simulink model "Copy_of_minimal_rcu_full"  (R2014b)
settings: Solver=ode4  SolverMode=SingleTasking  StartTime=0.0  StopTime=t_sim  FixedStep=sample_time_model  RelTol=1e-3
PreLoadFcn:
  | initModell
InitFcn:
  | initModell
undefined symbols (not defined in the file): FILTER_TAU_EXT, FIXED_FILTER_BANDWIDTH, FIXED_FILTER_BANDWIDTH_OBSERVER, iter, K_INV, KI2TAU_VEC, KS_trq, KT_trq, load_inertia, load_mass, MAX_CURRENT, MIN_SING_VALUE_M_CART, q0, rCEE_i, sample_time_model, sample_time_robot, tau_max
libraries: simulink x69, robotics x15, beasty_sfcns x7, lwr_dynamics x6, trafo3dLib x4, holgersRobLib x3, dspmtrx3 x1, dspinverses x1
(part 4 of 4)

== system Copy_of_minimal_rcu_full/Roboter+controller/controller/Cartesian Impedance Control/Subsystem/Cartesian Compliance Control/Iterative Computation of the 'Stiffness' and Gravity Compensation/Iteration for Nolcos Controller/Spatial Stiffness ==
  Hsd : Inport
  Fkin : Inport  Port=2
  Jbody : Inport  Port=3
  K : Inport  Port=4
  relaxing : Inport  Port=5
  Enable : EnablePort  StatesWhenEnabling=reset
  Kc : Selector  NumberOfDimensions=2  InputPortWidth=3  IndexOptions=Index vector (dialog),Index vector (dialog)  Indices=1:3,4:6
  Kr : Selector  NumberOfDimensions=2  InputPortWidth=3  IndexOptions=Index vector (dialog),Index vector (dialog)  Indices=4:6,4:6
  Kt : Selector  NumberOfDimensions=2  InputPortWidth=3  IndexOptions=Index vector (dialog),Index vector (dialog)  Indices=1:3,1:3
  Math Function : Math  Operator=transpose  SaturateOnIntegerOverflow=on
  Product2 : Product  RndMeth=Zero
  Product4 : Product  Multiplication=Matrix(*)  RndMeth=Zero
  Reshape1 : Reshape
  Reshape2 : Reshape
  Reshape3 : Reshape  OutputDimensionality=Column vector (2-D)
  Spatial Stiffness with varying length and varying stiffness : Subsystem  AncestorBlock=|
      | robotics/Spatial Stiffness
      | with varying length
      | and varying stiffness
  Terminator : Terminator
  Trafo3D Inverse : robotics/Trafo3D Inverse
  Trafo3D Mult : robotics/Trafo3D Mult
  unit frame : Constant  Value=[eye(3),[0;0;0]]
  tau : Outport
  J : Outport  Port=2
  F : Outport  Port=3
  wires:
  Product4/1 -> Reshape2/1
  Jbody/1 -> J/1, Math Function/1
  Math Function/1 -> Product4/1
  Hsd/1 -> Trafo3D Inverse/1
  Trafo3D Inverse/1 -> Trafo3D Mult/1
  Fkin/1 -> Trafo3D Mult/2
  Trafo3D Mult/1 -> Spatial Stiffness with varying length and varying stiffness/1(H12)
  unit frame/1 -> Spatial Stiffness with varying length and varying stiffness/2(H1,1c), Spatial Stiffness with varying length and varying stiffness/3(H2,2c)
  Spatial Stiffness with varying length and varying stiffness/2(W2) -> Product2/1, Reshape1/1
  K/1 -> Kt/1, Kr/1, Kc/1
  Kt/1 -> Spatial Stiffness with varying length and varying stiffness/4(Kt)
  Kr/1 -> Spatial Stiffness with varying length and varying stiffness/5(Kr)
  Kc/1 -> Spatial Stiffness with varying length and varying stiffness/6(Kc)
  relaxing/1 -> Reshape3/1
  Product2/1 -> Product4/2
  Spatial Stiffness with varying length and varying stiffness/1(W1) -> Terminator/1
  Reshape1/1 -> F/1
  Reshape2/1 -> tau/1
  Reshape3/1 -> Product2/2

== system Copy_of_minimal_rcu_full/Roboter+controller/controller/Cartesian Impedance Control/Subsystem/Cartesian Compliance Control/Nullspace Stiffness1/Stiffness Calculation/Calculate reflected Inertia ==
  B_JT_4 : Inport
  0_T_4 : Inport  Port=2
  Mass : Inport  Port=3
  Math Function1 : Math  Operator=transpose  SaturateOnIntegerOverflow=on
  Product : Product  Multiplication=Matrix(*)  RndMeth=Zero
  Product1 : Product  Inputs=3  Multiplication=Matrix(*)  RndMeth=Zero
  Selector translation1 : Selector  NumberOfDimensions=2  InputPortWidth=6  IndexOptions=Index vector (dialog),Index vector (dialog)  Indices=3,3  OutputSizes=1,1
  Trafo3D Adjoint : trafo3dLib/Trafo3D Adjoint
  m_z : Outport
  wires:
  Selector translation1/1 -> m_z/1
  Trafo3D Adjoint/1 -> Product/2
  Math Function1/1 -> Product1/1
  Product/1 -> Product1/3, Math Function1/1
  Product1/1 -> Selector translation1/1
  Mass/1 -> Product1/2
  B_JT_4/1 -> Product/1
  0_T_4/1 -> Trafo3D Adjoint/1

== system Copy_of_minimal_rcu_full/Roboter+controller/controller/Cartesian Impedance Control/Subsystem/Cartesian Compliance Control/Nullspace Stiffness1/Stiffness Calculation/Normalize Vector ==
  In1 : Inport
  Constant : Constant
  Demux : Demux  Outputs=[-1 1]
  Divide : Product  Inputs=*/
  Ground : Ground
  Math Function : Math  Operator=square  SaturateOnIntegerOverflow=on
  Math Function1 : Math  Operator=sqrt  SaturateOnIntegerOverflow=on
  Mux : Mux  Inputs=2
  Mux1 : Mux  Inputs=2
  Product : Product  RndMeth=Zero
  Sum of Elements : Sum  Inputs=+
  Switch : Switch  Criteria=u2 > Threshold  Threshold=maxzero
  Out1 : Outport
  wires:
  Ground/1 -> Product/2
  Product/1 -> Mux1/1
  Constant/1 -> Mux1/2
  Mux1/1 -> Switch/3
  Sum of Elements/1 -> Math Function1/1
  Math Function/1 -> Sum of Elements/1
  Demux/2 -> Divide/2
  Demux/1 -> Divide/1
  Switch/1 -> Demux/1
  Mux/1 -> Switch/1
  Math Function1/1 -> Mux/2, Switch/2
  In1/1 -> Product/1, Math Function/1, Mux/1
  Divide/1 -> Out1/1

== system Copy_of_minimal_rcu_full/Roboter+controller/controller/Cartesian Impedance Control/Subsystem/Cartesian Compliance Control/Nullspace Stiffness1/Stiffness Calculation/PT1_1 ==
  In1 : Inport
  Gain : Gain  Gain=3
  Integrator : Integrator  InitialCondition=[0 0 0]'
  Sum : Sum  Inputs=|+-
  Out1 : Outport  OutDataTypeStr=double  PortDimensions=[3 1]
  wires:
  Integrator/1 -> Sum/2, Out1/1
  Sum/1 -> Gain/1
  In1/1 -> Sum/1
  Gain/1 -> Integrator/1

== system Copy_of_minimal_rcu_full/Roboter+controller/controller/Cartesian Impedance Control/Subsystem/Cartesian Compliance Control/Nullspace Stiffness1/Stiffness Calculation/PT1_2 ==
  In1 : Inport
  Gain : Gain  Gain=3
  Integrator : Integrator
  Sum : Sum  Inputs=|+-
  Out1 : Outport  OutDataTypeStr=double  PortDimensions=1
  wires:
  Gain/1 -> Integrator/1
  In1/1 -> Sum/1
  Sum/1 -> Gain/1
  Integrator/1 -> Sum/2, Out1/1

== system Copy_of_minimal_rcu_full/Roboter+controller/controller/Joint Impedance/JOINT_IMPEDANCE_CONTROL/Joint Compliance Control/Damping Design via Generalized Eigenvalues/Damping Design via Generalized Eigenvalues QR right/Subsystem ==
  A : Inport
  B : Inport  Port=2
  Double diagonalization1 : MATLAB Function  TreatAsAtomicUnit=on
  V : Outport
  lambda : Outport  Port=2
  Vinv : Outport  Port=3
  wires:
  A/1 -> Double diagonalization1/1(A)
  B/1 -> Double diagonalization1/2(B)
  Double diagonalization1/3(lambda) -> lambda/1
  Double diagonalization1/2(Vinv) -> Vinv/1
  Double diagonalization1/1(V) -> V/1

== system Copy_of_minimal_rcu_full/Roboter+controller/controller/Cartesian Impedance Control/Subsystem/Cartesian Compliance Control/Iterative Computation of the 'Stiffness' and Gravity Compensation/Iteration for Nolcos Controller/Euler Angle Stiffness/Euler Angle Components ==
  Hsd : Inport
  Fkin : Inport  Port=2
  J : Inport  Port=3
  Cross-Product : robotics/Cross-Product
  Euler Transf. w->rpy' : robotics/Euler Transf. w->rpy'
  Jv : Selector  NumberOfDimensions=2  InputPortWidth=3  IndexOptions=Index vector (dialog),Select all  Indices=[1 2 3],-1
  Jw : Selector  NumberOfDimensions=2  InputPortWidth=3  IndexOptions=Index vector (dialog),Select all  Indices=[4 5 6],-1
  Matrix Concatenation1 : Concatenate  Mode=Multidimensional array
  Matrix Gain : Gain  Gain=-1  Multiplication=Matrix(K*u)  SaturateOnIntegerOverflow=on  OutDataTypeStr=Inherit: Same as input  ParamDataTypeStr=Inherit: Same as input
  Product1 : Product  Multiplication=Matrix(*)  RndMeth=Zero
  RPY Euler : robotics/RPY Euler  th=0.9999
  Stop Simulation1 : Stop
  Sum3 : Sum  Inputs=-+|  SaturateOnIntegerOverflow=on  InputSameDT=on  OutDataTypeStr=Inherit: Same as first input
  Trafo3D Inverse1 : robotics/Trafo3D Inverse
  Trafo3D Mult1 : robotics/Trafo3D Mult
  v : Selector  NumberOfDimensions=2  InputPortWidth=3  IndexOptions=Select all,Index vector (dialog)  Indices=-1,[4]
  x : Outport
  Jx : Outport  Port=2
  wires:
  Trafo3D Inverse1/1 -> Trafo3D Mult1/1
  Trafo3D Mult1/1 -> RPY Euler/1, v/1
  RPY Euler/2 -> Stop Simulation1/1
  RPY Euler/1 -> Euler Transf. w->rpy'/1, x/1
  v/1 -> Cross-Product/1
  Fkin/1 -> Trafo3D Inverse1/1
  Hsd/1 -> Trafo3D Mult1/2
  J/1 -> Jv/1, Jw/1
  Jw/1 -> Cross-Product/2, Matrix Gain/1
  Sum3/1 -> Matrix Concatenation1/1
  Cross-Product/1 -> Sum3/2
  Jv/1 -> Sum3/1
  Matrix Gain/1 -> Matrix Concatenation1/2
  Matrix Concatenation1/1 -> Product1/2
  Product1/1 -> Jx/1
  Euler Transf. w->rpy'/1 -> Product1/1

== system Copy_of_minimal_rcu_full/Roboter+controller/controller/Cartesian Impedance Control/Subsystem/Cartesian Compliance Control/Iterative Computation of the 'Stiffness' and Gravity Compensation/Iteration for Nolcos Controller/Spatial Stiffness/Spatial Stiffness with varying length and varying stiffness ==
  H12 : Inport
  H1,1c : Inport  Port=2
  H2,2c : Inport  Port=3
  Kt : Inport  Port=4
  Kr : Inport  Port=5
  Kc : Inport  Port=6
  Math Function : Math  Operator=transpose  SaturateOnIntegerOverflow=on
  Math Function1 : Math  Operator=transpose  SaturateOnIntegerOverflow=on
  Product : Product  Multiplication=Matrix(*)  RndMeth=Zero
  Product1 : Product  Multiplication=Matrix(*)  RndMeth=Zero
  Spatial Stiffness without connection offsets : Subsystem
  Trafo3D Adjoint : robotics/Trafo3D Adjoint
  Trafo3D Adjoint1 : robotics/Trafo3D Adjoint
  Trafo3D Inverse : robotics/Trafo3D Inverse
  Trafo3D Inverse1 : robotics/Trafo3D Inverse
  Trafo3D Mult : robotics/Trafo3D Mult
  Trafo3D Mult1 : robotics/Trafo3D Mult
  W1 : Outport
  W2 : Outport  Port=2
  wires:
  Kc/1 -> Spatial Stiffness without connection offsets/4(Kc)
  Kr/1 -> Spatial Stiffness without connection offsets/3(Kr)
  Kt/1 -> Spatial Stiffness without connection offsets/2(Kt)
  Product1/1 -> W2/1
  Spatial Stiffness without connection offsets/2(W2c) -> Product1/2
  Product/1 -> W1/1
  Spatial Stiffness without connection offsets/1(W1c) -> Product/2
  Trafo3D Mult1/1 -> Spatial Stiffness without connection offsets/1(H1c2c)
  H12/1 -> Trafo3D Mult/2
  Trafo3D Mult/1 -> Trafo3D Mult1/1
  Trafo3D Adjoint/1 -> Math Function/1  "AdH1c,1"
  Trafo3D Adjoint1/1 -> Math Function1/1  "AdH2c,2"
  Math Function/1 -> Product/1
  Math Function1/1 -> Product1/1
  H1,1c/1 -> Trafo3D Inverse/1
  Trafo3D Inverse/1 -> Trafo3D Mult/1, Trafo3D Adjoint/1  "H1c,1"
  H2,2c/1 -> Trafo3D Mult1/2, Trafo3D Inverse1/1
  Trafo3D Inverse1/1 -> Trafo3D Adjoint1/1

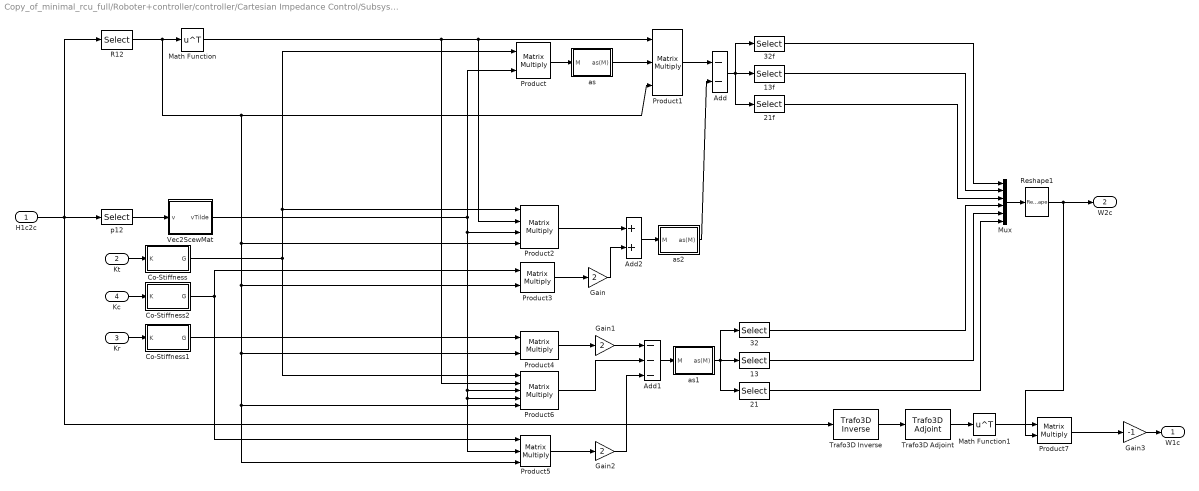
== system Copy_of_minimal_rcu_full/Roboter+controller/controller/Cartesian Impedance Control/Subsystem/Cartesian Compliance Control/Iterative Computation of the 'Stiffness' and Gravity Compensation/Iteration for Nolcos Controller/Spatial Stiffness/Spatial Stiffness with varying length and varying stiffness/Spatial Stiffness without connection offsets ==
  H1c2c : Inport
  Kt : Inport  Port=2
  Kr : Inport  Port=3
  Kc : Inport  Port=4
  13 : Selector  NumberOfDimensions=2  InputPortWidth=3  IndexOptions=Index vector (dialog),Index vector (dialog)  Indices=[1],[3]
  13f : Selector  NumberOfDimensions=2  InputPortWidth=3  IndexOptions=Index vector (dialog),Index vector (dialog)  Indices=[1],[3]
  21 : Selector  NumberOfDimensions=2  InputPortWidth=3  IndexOptions=Index vector (dialog),Index vector (dialog)  Indices=[2],[1]
  21f : Selector  NumberOfDimensions=2  InputPortWidth=3  IndexOptions=Index vector (dialog),Index vector (dialog)  Indices=[2],[1]
  32 : Selector  NumberOfDimensions=2  InputPortWidth=3  IndexOptions=Index vector (dialog),Index vector (dialog)  Indices=[3],[2]
  32f : Selector  NumberOfDimensions=2  InputPortWidth=3  IndexOptions=Index vector (dialog),Index vector (dialog)  Indices=[3],[2]
  Add : Sum  Inputs=--
  Add1 : Sum  Inputs=---
  Add2 : Sum
  Co-Stiffness : Subsystem
  Co-Stiffness1 : Subsystem
  Co-Stiffness2 : Subsystem
  Gain : Gain  Gain=2
  Gain1 : Gain  Gain=2
  Gain2 : Gain  Gain=2
  Gain3 : Gain  Gain=-1
  Math Function : Math  Operator=transpose  SaturateOnIntegerOverflow=on
  Math Function1 : Math  Operator=transpose  SaturateOnIntegerOverflow=on
  Mux : Mux  Inputs=6
  Product{,3..4,7} (4 alike) : Product  Multiplication=Matrix(*)  SaturateOnIntegerOverflow=on  InputSameDT=on  OutDataTypeStr=Inherit: Same as first input
  Product1 : Product  Inputs=3  Multiplication=Matrix(*)  SaturateOnIntegerOverflow=on  InputSameDT=on  OutDataTypeStr=Inherit: Same as first input
  Product2 : Product  Inputs=4  Multiplication=Matrix(*)  SaturateOnIntegerOverflow=on  InputSameDT=on  OutDataTypeStr=Inherit: Same as first input
  Product5 : Product  Inputs=3  Multiplication=Matrix(*)  SaturateOnIntegerOverflow=on  InputSameDT=on  OutDataTypeStr=Inherit: Same as first input
  Product6 : Product  Inputs=5  Multiplication=Matrix(*)  SaturateOnIntegerOverflow=on  InputSameDT=on  OutDataTypeStr=Inherit: Same as first input
  R12 : Selector  NumberOfDimensions=2  InputPortWidth=3  IndexOptions=Index vector (dialog),Index vector (dialog)  Indices=[1,2,3],[1,2,3]
  Reshape1 : Reshape  OutputDimensionality=Column vector (2-D)
  Trafo3D Adjoint : robotics/Trafo3D Adjoint
  Trafo3D Inverse : robotics/Trafo3D Inverse
  Vec2ScewMat : Subsystem
  as : Subsystem
  as1 : Subsystem
  as2 : Subsystem
  p12 : Selector  NumberOfDimensions=2  InputPortWidth=3  IndexOptions=Index vector (dialog),Index vector (dialog)  Indices=[1,2,3],[4]
  W1c : Outport
  W2c : Outport  Port=2
  wires:
  H1c2c/1 -> p12/1, R12/1, Trafo3D Inverse/1
  Kc/1 -> Co-Stiffness2/1(K)
  Kr/1 -> Co-Stiffness1/1(K)
  Kt/1 -> Co-Stiffness/1(K)
  Math Function1/1 -> Product7/1
  Trafo3D Adjoint/1 -> Math Function1/1
  Gain3/1 -> W1c/1
  Product7/1 -> Gain3/1
  Trafo3D Inverse/1 -> Trafo3D Adjoint/1
  21/1 -> Mux/6
  13/1 -> Mux/5
  32/1 -> Mux/4
  21f/1 -> Mux/3
  13f/1 -> Mux/2
  32f/1 -> Mux/1
  Add/1 -> 21f/1, 32f/1, 13f/1
  as1/1(as(M)) -> 21/1, 13/1, 32/1
  Gain2/1 -> Add1/3
  Gain1/1 -> Add1/1
  Product6/1 -> Add1/2
  Product5/1 -> Gain2/1
  Add1/1 -> as1/1(M)
  as2/1(as(M)) -> Add/2
  Add2/1 -> as2/1(M)
  Gain/1 -> Add2/2
  Product2/1 -> Add2/1
  Co-Stiffness1/1(G) -> Product4/1
  Product4/1 -> Gain1/1
  Mux/1 -> Reshape1/1
  Co-Stiffness2/1(G) -> Product5/1, Product3/1
  Product3/1 -> Gain/1
  Product1/1 -> Add/1
  Math Function/1 -> Product6/2, Product2/2, Product1/1
  R12/1 -> Math Function/1, Product5/3, Product6/5, Product4/2, Product3/2, Product2/4, Product1/3
  as/1(as(M)) -> Product1/2
  Product/1 -> as/1(M)
  Vec2ScewMat/1(vTilde) -> Product5/2, Product6/4, Product6/3, Product2/3, Product/2
  Co-Stiffness/1(G) -> Product6/1, Product2/1, Product/1
  p12/1 -> Vec2ScewMat/1(v)
  Reshape1/1 -> W2c/1, Product7/2

== system Copy_of_minimal_rcu_full/Roboter+controller/controller/Cartesian Impedance Control/Subsystem/Cartesian Compliance Control/Iterative Computation of the 'Stiffness' and Gravity Compensation/Iteration for Nolcos Controller/Spatial Stiffness/Spatial Stiffness with varying length and varying stiffness/Spatial Stiffness without connection offsets/Co-Stiffness ==
  K : Inport
  Add1 : Sum  Inputs=|+-
  Add2 : Sum  Inputs=+++
  Gain3 : Gain  Gain=0.5
  K11 : Selector  NumberOfDimensions=2  InputPortWidth=3  IndexOptions=Index vector (dialog),Index vector (dialog)  Indices=1,1
  K22 : Selector  NumberOfDimensions=2  InputPortWidth=3  IndexOptions=Index vector (dialog),Index vector (dialog)  Indices=2,2
  K33 : Selector  NumberOfDimensions=2  InputPortWidth=3  IndexOptions=Index vector (dialog),Index vector (dialog)  Indices=3,3
  Product1 : Product  SaturateOnIntegerOverflow=on  InputSameDT=on  OutDataTypeStr=Inherit: Same as first input
  eye : Constant  Value=eye(3)
  G : Outport
  wires:
  Add1/1 -> G/1
  Gain3/1 -> Add1/1
  Product1/1 -> Gain3/1
  eye/1 -> Product1/2
  Add2/1 -> Product1/1
  K33/1 -> Add2/3
  K11/1 -> Add2/1
  K22/1 -> Add2/2
  K/1 -> Add1/2, K33/1, K22/1, K11/1

== system Copy_of_minimal_rcu_full/Roboter+controller/controller/Cartesian Impedance Control/Subsystem/Cartesian Compliance Control/Iterative Computation of the 'Stiffness' and Gravity Compensation/Iteration for Nolcos Controller/Spatial Stiffness/Spatial Stiffness with varying length and varying stiffness/Spatial Stiffness without connection offsets/Co-Stiffness1 ==
  K : Inport
  Add1 : Sum  Inputs=|+-
  Add2 : Sum  Inputs=+++
  Gain3 : Gain  Gain=0.5
  K11 : Selector  NumberOfDimensions=2  InputPortWidth=3  IndexOptions=Index vector (dialog),Index vector (dialog)  Indices=1,1
  K22 : Selector  NumberOfDimensions=2  InputPortWidth=3  IndexOptions=Index vector (dialog),Index vector (dialog)  Indices=2,2
  K33 : Selector  NumberOfDimensions=2  InputPortWidth=3  IndexOptions=Index vector (dialog),Index vector (dialog)  Indices=3,3
  Product1 : Product  SaturateOnIntegerOverflow=on  InputSameDT=on  OutDataTypeStr=Inherit: Same as first input
  eye : Constant  Value=eye(3)
  G : Outport
  wires:
  K/1 -> K11/1, K22/1, K33/1, Add1/2
  K22/1 -> Add2/2
  K11/1 -> Add2/1
  K33/1 -> Add2/3
  Add2/1 -> Product1/1
  eye/1 -> Product1/2
  Product1/1 -> Gain3/1
  Gain3/1 -> Add1/1
  Add1/1 -> G/1

== system Copy_of_minimal_rcu_full/Roboter+controller/controller/Cartesian Impedance Control/Subsystem/Cartesian Compliance Control/Iterative Computation of the 'Stiffness' and Gravity Compensation/Iteration for Nolcos Controller/Spatial Stiffness/Spatial Stiffness with varying length and varying stiffness/Spatial Stiffness without connection offsets/Co-Stiffness2 ==
  K : Inport
  Add1 : Sum  Inputs=|+-
  Add2 : Sum  Inputs=+++
  Gain3 : Gain  Gain=0.5
  K11 : Selector  NumberOfDimensions=2  InputPortWidth=3  IndexOptions=Index vector (dialog),Index vector (dialog)  Indices=1,1
  K22 : Selector  NumberOfDimensions=2  InputPortWidth=3  IndexOptions=Index vector (dialog),Index vector (dialog)  Indices=2,2
  K33 : Selector  NumberOfDimensions=2  InputPortWidth=3  IndexOptions=Index vector (dialog),Index vector (dialog)  Indices=3,3
  Product1 : Product  SaturateOnIntegerOverflow=on  InputSameDT=on  OutDataTypeStr=Inherit: Same as first input
  eye : Constant  Value=eye(3)
  G : Outport
  wires:
  Add1/1 -> G/1
  Gain3/1 -> Add1/1
  Product1/1 -> Gain3/1
  eye/1 -> Product1/2
  Add2/1 -> Product1/1
  K33/1 -> Add2/3
  K11/1 -> Add2/1
  K22/1 -> Add2/2
  K/1 -> Add1/2, K33/1, K22/1, K11/1

== system Copy_of_minimal_rcu_full/Roboter+controller/controller/Cartesian Impedance Control/Subsystem/Cartesian Compliance Control/Iterative Computation of the 'Stiffness' and Gravity Compensation/Iteration for Nolcos Controller/Spatial Stiffness/Spatial Stiffness with varying length and varying stiffness/Spatial Stiffness without connection offsets/Vec2ScewMat ==
  v : Inport
  Gain : Gain  Gain=-1  SaturateOnIntegerOverflow=on  OutDataTypeStr=Inherit: Same as input  ParamDataTypeStr=Inherit: Same as input
  Gain1 : Gain  Gain=-1  SaturateOnIntegerOverflow=on  OutDataTypeStr=Inherit: Same as input  ParamDataTypeStr=Inherit: Same as input
  Gain2 : Gain  Gain=-1  SaturateOnIntegerOverflow=on  OutDataTypeStr=Inherit: Same as input  ParamDataTypeStr=Inherit: Same as input
  Matrix Concatenation1 : Concatenate  NumInputs=3  Mode=Multidimensional array
  Matrix Concatenation2 : Concatenate  NumInputs=3  Mode=Multidimensional array
  Matrix Concatenation3 : Concatenate  NumInputs=3  Mode=Multidimensional array
  Matrix Concatenation4 : Concatenate  NumInputs=3  Mode=Multidimensional array  ConcatenateDimension=2
  Selector : Selector  InputPortWidth=3  Indices=[1]
  Selector1 : Selector  InputPortWidth=3  Indices=[2]
  Selector2 : Selector  InputPortWidth=3  Indices=[3]
  zero : Constant  Value=0
  vTilde : Outport
  wires:
  Matrix Concatenation4/1 -> vTilde/1
  zero/1 -> Matrix Concatenation2/1, Matrix Concatenation1/2, Matrix Concatenation3/3
  Selector/1 -> Gain/1, Matrix Concatenation1/3
  Selector1/1 -> Gain1/1, Matrix Concatenation3/1
  Selector2/1 -> Gain2/1, Matrix Concatenation2/2
  Gain1/1 -> Matrix Concatenation2/3
  Gain2/1 -> Matrix Concatenation1/1
  Matrix Concatenation2/1 -> Matrix Concatenation4/1
  Matrix Concatenation1/1 -> Matrix Concatenation4/2
  Matrix Concatenation3/1 -> Matrix Concatenation4/3
  Gain/1 -> Matrix Concatenation3/2
  v/1 -> Selector/1, Selector1/1, Selector2/1

== system Copy_of_minimal_rcu_full/Roboter+controller/controller/Cartesian Impedance Control/Subsystem/Cartesian Compliance Control/Iterative Computation of the 'Stiffness' and Gravity Compensation/Iteration for Nolcos Controller/Spatial Stiffness/Spatial Stiffness with varying length and varying stiffness/Spatial Stiffness without connection offsets/as ==
  M : Inport
  Add : Sum  Inputs=+-
  Gain : Gain  Gain=0.5
  Math Function : Math  Operator=transpose  SaturateOnIntegerOverflow=on
  as(M) : Outport
  wires:
  Add/1 -> Gain/1
  Math Function/1 -> Add/2
  M/1 -> Add/1, Math Function/1
  Gain/1 -> as(M)/1

== system Copy_of_minimal_rcu_full/Roboter+controller/controller/Cartesian Impedance Control/Subsystem/Cartesian Compliance Control/Iterative Computation of the 'Stiffness' and Gravity Compensation/Iteration for Nolcos Controller/Spatial Stiffness/Spatial Stiffness with varying length and varying stiffness/Spatial Stiffness without connection offsets/as1 ==
  M : Inport
  Add : Sum  Inputs=+-
  Gain : Gain  Gain=0.5
  Math Function : Math  Operator=transpose  SaturateOnIntegerOverflow=on
  as(M) : Outport
  wires:
  Gain/1 -> as(M)/1
  M/1 -> Add/1, Math Function/1
  Math Function/1 -> Add/2
  Add/1 -> Gain/1

== system Copy_of_minimal_rcu_full/Roboter+controller/controller/Cartesian Impedance Control/Subsystem/Cartesian Compliance Control/Iterative Computation of the 'Stiffness' and Gravity Compensation/Iteration for Nolcos Controller/Spatial Stiffness/Spatial Stiffness with varying length and varying stiffness/Spatial Stiffness without connection offsets/as2 ==
  M : Inport
  Add : Sum  Inputs=+-
  Gain : Gain  Gain=0.5
  Math Function : Math  Operator=transpose  SaturateOnIntegerOverflow=on
  as(M) : Outport
  wires:
  Add/1 -> Gain/1
  Math Function/1 -> Add/2
  M/1 -> Add/1, Math Function/1
  Gain/1 -> as(M)/1

== matlab function Copy_of_minimal_rcu_full/Roboter+controller/controller/Cartesian Impedance Control/Subsystem/Cartesian Compliance Control/cmd2/Embedded MATLAB Function1 ==
  settings: fimath=|
      | fimath(...
      | 'RoundMode', 'floor',...
      | 'OverflowMode', 'wrap',...
      | 'ProductMode', 'KeepLSB', 'ProductWordLength', 32,...
      | 'SumMode', 'KeepLSB', 'SumWordLength', 32,...
      | 'CastBeforeSum', false)
  data: K_diag input; K output; K_sqrt output
function [K, K_sqrt]  = mystiffness(K_diag)
% This block supports an embeddable subset of the MATLAB language.
% See the help menu for details. 

K = diag(K_diag);
K_sqrt = sqrt(K);

== matlab function Copy_of_minimal_rcu_full/Roboter+controller/controller/Cartesian Impedance Control/Subsystem/Cartesian Compliance Control/Cartesian Damping/Cartesian mass matrix/Subsystem1/inv with hold ==
  settings: fimath=|
      | fimath(...
      | 'RoundMode', 'floor',...
      | 'OverflowMode', 'wrap',...
      | 'ProductMode', 'KeepLSB', 'ProductWordLength', 32,...
      | 'SumMode', 'KeepLSB', 'SumWordLength', 32,...
      | 'CastBeforeSum', false)
  data: not_singular output; inv_matrix output size=[6,6]; in_matrix input; min_singular_value input; inv_matrix_sqrt output
function [not_singular, inv_matrix, inv_matrix_sqrt ]= inverse_with_hold( in_matrix, min_singular_value)
% WARNING: works only for symetric, positive semidefinite matrices 

[u, s, v] = svd(in_matrix);
s_diag = diag(s);
%if( min(s_diag) < min_singular_value )
%    out_matrix = valid_out_matrix;
%    not_singular = 0;
%else
%    s_inv = 1./s_diag; 
%    out_matrix = u*diag(s_inv)*v';
%    not_singular = 1;
%    valid_out_matrix = out_matrix;
%end



if( min(s_diag) < min_singular_value )
     %s_diag(find(s_diag<min_singular_value))= min_singular_value
     for i=1:1:length(s_diag)
         if s_diag(i) < min_singular_value
             s_diag(i) = min_singular_value;
         end
     end
     not_singular = 0;
else
     not_singular = 1;
end


s_inv = 1./s_diag; 
s_inv_sqrt =sqrt(s_inv);
inv_matrix = u*diag(s_inv)*u';   % you can use u instead of v because the matrix is p.s.d.
inv_matrix_sqrt = u*diag(s_inv_sqrt)*u';

== matlab function Copy_of_minimal_rcu_full/Roboter+controller/controller/Joint Impedance/JOINT_IMPEDANCE_CONTROL/Joint Compliance Control/Damping Design via Generalized Eigenvalues/Damping Design via Generalized Eigenvalues QR right/Subsystem/Double diagonalization1 ==
  data: V output; A input; B input; Vinv output; lambda output
function [V, Vinv, lambda] = fcn(A,B)

% if the matrices are symmetric and p.d., both Vc and Lambda are real
[Vc, Lambda] = eig(A,B);
lambda=real(diag(Lambda));
V=real(Vc);
Vinv=inv(V);

== matlab function Copy_of_minimal_rcu_full/Roboter+controller/controller/Cartesian Impedance Control/calculate Feedforward/check if  matrix  is SO(3) ==
  data: matrix input; EE_T_K output
function EE_T_K = fcn(matrix)

EE_T_K = matrix;

determinant = det(matrix(1:3,1:3));
if (determinant < 0.9 || determinant > 1.1)
    EE_T_K = eye(4,4);
end

== matlab function Copy_of_minimal_rcu_full/Roboter+controller/controller/Cartesian Impedance Control/calculate Feedforward/check if  matrix  is SO(3)1 ==
  data: matrix input; TCP_T_EE output
function TCP_T_EE = fcn(matrix)

TCP_T_EE = matrix;

determinant = det(matrix(1:3,1:3));
if (determinant < 0.9 || determinant > 1.1)
    TCP_T_EE = eye(4,4);
end

== matlab function Copy_of_minimal_rcu_full/Roboter+controller/controller/Cartesian Impedance Control/Subsystem/Cartesian Compliance Control/Singularity Avoidance/Proj. ==
  settings: fimath=|
      | fimath(...
      | 'RoundMode', 'floor',...
      | 'OverflowMode', 'wrap',...
      | 'ProductMode', 'KeepLSB', 'ProductWordLength', 32,...
      | 'SumMode', 'KeepLSB', 'SumWordLength', 32,...
      | 'CastBeforeSum', false)
  data: tau input; P output
function P = fcn(tau)
% This block supports an embeddable subset of the MATLAB language.
% See the help menu for details. 

P = tau*pinv(tau);

== stateflow chart Copy_of_minimal_rcu_full/Roboter+controller/controller/Joint Impedance/JOINT_IMPEDANCE_CONTROL/Joint Compliance Control/NAN_checks/hold_zero_if_nan_or_inf1/Hold1 ==
  settings: executeAtInitialization=1
  state OK
    en:error=0;
  state FAIL
    en:error=1;
  (default) -> OK
  OK -> FAIL : isnan
  FAIL -> OK : reset
  data: error output double
  events: isnan input RISING_EDGE_EVENT; reset input RISING_EDGE_EVENT

== matlab function Copy_of_minimal_rcu_full/Roboter+controller/controller/Cartesian Impedance Control/Subsystem/Cartesian Compliance Control/Cartesian Damping/Damping Design via Generalized Eigenvalues/Damping Design via Generalized Eigenvalues QR right/Double diagonalization ==
  data: A input; V output; Vinv output; B input; lambda output
function [V, Vinv, lambda] = fcn(A,B)
% This block supports an embeddable subset of the MATLAB language.
% See the help menu for details. 


% if the matrices are symmetric and p.d., both Vc and Lambda are real
[Vc, Lambda] = eig(A,B);
lambda=real(diag(Lambda));
V=real(Vc);
Vinv=inv(V);

== matlab function Copy_of_minimal_rcu_full/Roboter+controller/controller/Joint Impedance/JOINT_IMPEDANCE_CONTROL/Joint Compliance Control/Embedded MATLAB Function ==
  settings: fimath=|
      | fimath(...
      | 'RoundMode', 'floor',...
      | 'OverflowMode', 'wrap',...
      | 'ProductMode', 'KeepLSB', 'ProductWordLength', 32,...
      | 'SumMode', 'KeepLSB', 'SumWordLength', 32,...
      | 'CastBeforeSum', false)
  data: u input; y output
function y = mydiag(u)
% This block supports an embeddable subset of the MATLAB language.
% See the help menu for details. 

y = diag(u);

== matlab function Copy_of_minimal_rcu_full/Roboter+controller/controller/Joint Impedance/JOINT_IMPEDANCE_CONTROL/Joint Compliance Control/Pragmatic Solution/Stiffness correction ==
  settings: fimath=|
      | fimath(...
      | 'RoundMode', 'floor',...
      | 'OverflowMode', 'wrap',...
      | 'ProductMode', 'KeepLSB', 'ProductWordLength', 32,...
      | 'SumMode', 'KeepLSB', 'SumWordLength', 32,...
      | 'CastBeforeSum', false)
  data: Kdes input; Kcontrol output
function Kcontrol = fcn(Kdes)

Kcontrol = 1000* [6.9000,10.8547,10.0000,10.0000,6.4643,10.0000,10.0000]';

for kk=1:7,
    if Kdes(kk)<Kcontrol(kk)*0.95,  % allow maximum 95% of joint stiffness
        Kcontrol(kk) = 1/(1/Kdes(kk)-1/Kcontrol(kk));
    end
end

== matlab function Copy_of_minimal_rcu_full/Roboter+controller/controller/Cartesian Impedance Control/Subsystem/Cartesian Compliance Control/Cartesian Damping/Damping_design/Embedded MATLAB Function1 ==
  settings: fimath=|
      | fimath(...
      | 'RoundMode', 'floor',...
      | 'OverflowMode', 'wrap',...
      | 'ProductMode', 'KeepLSB', 'ProductWordLength', 32,...
      | 'SumMode', 'KeepLSB', 'SumWordLength', 32,...
      | 'CastBeforeSum', false)
  data: u input; y output
function y = mydiag(u)
% This block supports an embeddable subset of the MATLAB language.
% See the help menu for details. 

y = diag(u);

== matlab function Copy_of_minimal_rcu_full/Roboter+controller/controller/Cartesian Impedance Control/Subsystem/Cartesian Compliance Control/cmd/Embedded MATLAB Function1 ==
  settings: fimath=|
      | fimath(...
      | 'RoundMode', 'floor',...
      | 'OverflowMode', 'wrap',...
      | 'ProductMode', 'KeepLSB', 'ProductWordLength', 32,...
      | 'SumMode', 'KeepLSB', 'SumWordLength', 32,...
      | 'CastBeforeSum', false)
  data: K_diag input; K output
function K  = mystiffness(K_diag)
% This block supports an embeddable subset of the MATLAB language.
% See the help menu for details. 

K = diag(K_diag);

== matlab function Copy_of_minimal_rcu_full/Roboter+controller/controller/Cartesian Impedance Control/Subsystem/Cartesian Compliance Control/Cartesian Damping/Damping Design via Generalized Eigenvalues/Damping Design via Generalized Eigenvalues QR right/Embedded MATLAB Function ==
  settings: fimath=|
      | fimath(...
      | 'RoundMode', 'floor',...
      | 'OverflowMode', 'wrap',...
      | 'ProductMode', 'KeepLSB', 'ProductWordLength', 32,...
      | 'SumMode', 'KeepLSB', 'SumWordLength', 32,...
      | 'CastBeforeSum', false)
  data: u input; y output
function y = fcn(u)
% This block supports an embeddable subset of the MATLAB language.
% See the help menu for details. 

y = diag(u);

== matlab function Copy_of_minimal_rcu_full/Roboter+controller/controller/Joint Impedance/JOINT_IMPEDANCE_CONTROL/Joint Compliance Control/Damping Design via Generalized Eigenvalues/Damping Design via Generalized Eigenvalues QR right/Embedded MATLAB Function ==
  settings: fimath=|
      | fimath(...
      | 'RoundMode', 'floor',...
      | 'OverflowMode', 'wrap',...
      | 'ProductMode', 'KeepLSB', 'ProductWordLength', 32,...
      | 'SumMode', 'KeepLSB', 'SumWordLength', 32,...
      | 'CastBeforeSum', false)
  data: u input; y output
function y = fcn(u)
% This block supports an embeddable subset of the MATLAB language.
% See the help menu for details. 

y = diag(u);

== matlab function Copy_of_minimal_rcu_full/Ipol/joint_ipol_5th_traj_scaling/Subsystem/Cartesian_ipol1/translation/Embedded MATLAB Function ==
  settings: fimath=|
      | fimath(...
      | 'RoundMode', 'floor',...
      | 'OverflowMode', 'wrap',...
      | 'ProductMode', 'KeepLSB', 'ProductWordLength', 32,...
      | 'SumMode', 'KeepLSB', 'SumWordLength', 32,...
      | 'CastBeforeSum', false)
  data: i output; delta input; maximum output
function [i, maximum] = fcn(delta)
% This block supports an embeddable subset of the MATLAB language.
% See the help menu for details. 

[maximum i] = max(delta);
i = min(i); % Falls gleicher Abstand fuer mindestens zwei der delta_i

== matlab function Copy_of_minimal_rcu_full/Ipol/joint_ipol_5th_traj_scaling/Subsystem/Cartesian_ipol1/translation/Embedded MATLAB Function1 ==
  settings: fimath=|
      | fimath(...
      | 'RoundMode', 'floor',...
      | 'OverflowMode', 'wrap',...
      | 'ProductMode', 'KeepLSB', 'ProductWordLength', 32,...
      | 'SumMode', 'KeepLSB', 'SumWordLength', 32,...
      | 'CastBeforeSum', false)
  data: t input; qd output; s0 input; v0 input; sf input; vm input; am input; dqd output; ddqd output; ipol_finished output
function [qd,dqd,ddqd, ipol_finished] = calc_qd(t,s0,v0,sf,vm,am)
    qd = 0;
    dqd = 0;
    ddqd = 0;
    
    parameters = zeros(15,1);
    parameters=compute_traj_parameters(s0, v0, sf, vm, am);
    [ipol_finished tmp] =interpolator(t, parameters);
    if sf==s0
        qd = s0;
        dqd = v0;
        ddqd= 0;
    else
        qd = tmp(1);
        dqd = tmp(2);
        ddqd = tmp(3);        
    end
end

function ris=compute_traj_parameters(s0, v0, sf, vm, am)
    ris=zeros(15,1);
    radix=zeros(2,1);
    T1 = 0;
    dT = 0;
    T2 = 0;
    a1 = 0;
    b1 = 0;
    c1 = 0;
    d1 = 0;
    e1 = 0;
    a2 = 0;
    b2 = 0;
    c2 = 0;
    d2 = 0;
    e2 = 0;
    k = 0;

    if (vm~=0) %check...
        vm=vm*sign(sf-s0);
        k=am*sign(sf-s0);
        T1 = -3/2*(v0-vm)/k;
        a1 = -4/27*k^3/(v0-vm)^2;
        b1 = -4/9*k^2/(v0-vm);
        e1 = s0;
        d1 = v0;
        c1 = 0;
        c2 = 0;
        T2 = 3/2*vm/k;
        dT = 1/4*(-3*vm^2+4*sf*k-4*a1*T1^4*k-4*b1*T1^3*k-4*c1*T1^2*k-4*d1*T1*k-4*e1*k)/vm/k;
        a2 = 4/27*k^3/vm^2;
        d2 = vm;
        e2 = 1/4*(-3*vm^2+4*sf*k)/k;
        b2 = -4/9*k^2/vm;
        if (dT<0)
            c2 = 0;
            c1 = 0;
            a=2;
            b=12*v0;
            c=9*v0^2-12*sf*k+12*s0*k;
            radix(1)=(-b + sqrt(b^2-4*a*c))/(2*a);
            radix(2)=(-b - sqrt(b^2-4*a*c))/(2*a);
            %decide the correct root
            T1_a = 1/2*radix(1)/k;
            T2_a = 1/2*(radix(1)+3*v0)/k;
            T1_b = 1/2*radix(2)/k;
            T2_b = 1/2*(radix(2)+3*v0)/k;
                if (and(T1_a>=0, T2_a>=0))
                    r=radix(1);
                    T1=T1_a;
                    T2=T2_a;
                    dT=0;
                    two_phases=1;
                elseif (and(T1_b>=0, T2_b>=0))
                    r=radix(2);
                    T1=T1_b;
                    T2=T2_b;
                    dT=0;
                    two_phases=1;
                else
                    r=0;
                    two_phases=0;
                end
                if (two_phases==0)
                    T1=0;
                    T2=2*(sf-s0)/v0;
                    dT=0;
                    b2=-1/4*v0^3/(sf-s0)^2;
                    c2=0;
                    a2=1/16*v0^4/(sf-s0)^3;
                    d2=v0;
                    e2=s0;
                else
                    b1 = -8/9*k^2/(4*v0*r+3*v0^2-4*sf*k+4*s0*k)*r;
                    a1 = 8/9*k^3/(4*v0*r+3*v0^2-4*sf*k+4*s0*k);
                    b2 = -8/9*k^2/(4*sf*k+3*v0^2-4*s0*k)*(r+3*v0);
                    e2 = -1/8*(3*v0^2-4*s0*k-4*sf*k)/k;
                    e1 = s0;
                    d1 = v0;
                    d2 = 2/9/(4*sf*k+3*v0^2-4*s0*k)*(r+3*v0)^3;
                    a2 = 8/9*k^3/(4*sf*k+3*v0^2-4*s0*k);
                end
        end
    end
    ris=[T1;dT;T2; a1; b1; c1; d1; e1; a2; b2; c2; d2; e2; vm; k];
end




%time, and the output of the previous function

function [ipol_finished ris]=interpolator(t, parameters)

ris=zeros(4,1);
T1=parameters(1);
dT=parameters(2);
T2=parameters(3);
a1=parameters(4);
b1=parameters(5);
c1=parameters(6);
d1=parameters(7);
e1=parameters(8);
a2=parameters(9);
b2=parameters(10);
c2=parameters(11);
d2=parameters(12);
e2=parameters(13);
vm=parameters(14);
k=parameters(15);


ipol_finished = 0;
if (vm~=0) %check...
        if (t<=T1)
            ris=[a1*t^4+b1*t^3+c1*t^2+d1*t+e1; 4*a1*t^3+3*b1*t^2+2*c1*t+d1; 12*a1*t^2+6*b1*t+2*c1; 1];
        elseif (t<=T1+dT)
            t=t-T1;
            ris=[a1*T1^4+b1*T1^3+c1*T1^2+d1*T1+e1+vm*t; vm; 0; 1];
        elseif (t<=T1+dT+T2)
            t=t-T1-dT;
            ris=[a2*t^4+b2*t^3+c2*t^2+d2*t+e2; 4*a2*t^3+3*b2*t^2+2*c2*t+d2; 12*a2*t^2+6*b2*t+2*c2; 1];
        else
            t=T2;
            ris=[a2*t^4+b2*t^3+c2*t^2+d2*t+e2;0;0; 0];
            ipol_finished=1;
        end
else
    ris=[0;0;0;1];
end

end

== matlab function Copy_of_minimal_rcu_full/Ipol/joint_ipol_5th_traj_scaling/Subsystem/Cartesian_ipol1/translation/Embedded MATLAB Function2 ==
  settings: fimath=|
      | fimath(...
      | 'RoundMode', 'floor',...
      | 'OverflowMode', 'wrap',...
      | 'ProductMode', 'KeepLSB', 'ProductWordLength', 32,...
      | 'SumMode', 'KeepLSB', 'SumWordLength', 32,...
      | 'CastBeforeSum', false)
  data: s0_q input; sf_q input; s0 output; i input; sf output
function [s0,sf] = fcn(s0_q, sf_q,i)
% This block supports an embeddable subset of the MATLAB language.
% See the help menu for details. 

s0 = s0_q(i);
sf = sf_q(i);

== matlab function Copy_of_minimal_rcu_full/Roboter+controller/controller/Cartesian Impedance Control/Subsystem/Cartesian Compliance Control/Nullspace Proj. ==
  settings: fimath=|
      | fimath(...
      | 'RoundMode', 'floor',...
      | 'OverflowMode', 'wrap',...
      | 'ProductMode', 'KeepLSB', 'ProductWordLength', 32,...
      | 'SumMode', 'KeepLSB', 'SumWordLength', 32,...
      | 'CastBeforeSum', false)
  data: J input; N output
function N = fcn(J)
% This block supports an embeddable subset of the MATLAB language.
% See the help menu for details. 

N = eye(7,7)-J'*pinv(J)';

== stateflow chart Copy_of_minimal_rcu_full/Roboter+controller/controller/Joint Impedance/JOINT_IMPEDANCE_CONTROL/Joint Compliance Control/NAN_checks/hold_zero_if_nan_or_inf2/Hold1 ==
  settings: executeAtInitialization=1
  state OK
    en:error=0;
  state FAIL
    en:error=1;
  (default) -> OK
  OK -> FAIL : isnan
  FAIL -> OK : reset
  data: error output double
  events: isnan input RISING_EDGE_EVENT; reset input RISING_EDGE_EVENT

== stateflow chart Copy_of_minimal_rcu_full/Roboter+controller/controller/Joint Impedance/JOINT_IMPEDANCE_CONTROL/Joint Compliance Control/NAN_checks/hold_zero_if_nan_or_inf3/Hold1 ==
  settings: executeAtInitialization=1
  state OK
    en:error=0;
  state FAIL
    en:error=1;
  (default) -> OK
  OK -> FAIL : isnan
  FAIL -> OK : reset
  data: error output double
  events: isnan input RISING_EDGE_EVENT; reset input RISING_EDGE_EVENT

== stateflow chart Copy_of_minimal_rcu_full/Roboter+controller/controller/Joint Impedance/JOINT_IMPEDANCE_CONTROL/Joint Compliance Control/NAN_checks/hold_zero_if_nan_or_inf4/Hold1 ==
  settings: executeAtInitialization=1
  state OK
    en:error=0;
  state FAIL
    en:error=1;
  (default) -> OK
  OK -> FAIL : isnan
  FAIL -> OK : reset
  data: error output double
  events: isnan input RISING_EDGE_EVENT; reset input RISING_EDGE_EVENT

== stateflow chart Copy_of_minimal_rcu_full/Roboter+controller/controller/Joint Impedance/JOINT_IMPEDANCE_CONTROL/Joint Compliance Control/NAN_checks/hold_zero_if_nan_or_inf5/Hold1 ==
  settings: executeAtInitialization=1
  state OK
    en:error=0;
  state FAIL
    en:error=1;
  (default) -> OK
  OK -> FAIL : isnan
  FAIL -> OK : reset
  data: error output double
  events: isnan input RISING_EDGE_EVENT; reset input RISING_EDGE_EVENT

== stateflow chart Copy_of_minimal_rcu_full/Roboter+controller/controller/Joint Impedance/JOINT_IMPEDANCE_CONTROL/Joint Compliance Control/NAN_checks/hold_zero_if_nan_or_inf6/Hold1 ==
  settings: executeAtInitialization=1
  state OK
    en:error=0;
  state FAIL
    en:error=1;
  (default) -> OK
  OK -> FAIL : isnan
  FAIL -> OK : reset
  data: error output double
  events: isnan input RISING_EDGE_EVENT; reset input RISING_EDGE_EVENT

== stateflow chart Copy_of_minimal_rcu_full/Roboter+controller/controller/Joint Impedance/JOINT_IMPEDANCE_CONTROL/Joint Compliance Control/NAN_checks/hold_zero_if_nan_or_inf7/Hold1 ==
  settings: executeAtInitialization=1
  state OK
    en:error=0;
  state FAIL
    en:error=1;
  (default) -> OK
  OK -> FAIL : isnan
  FAIL -> OK : reset
  data: error output double
  events: isnan input RISING_EDGE_EVENT; reset input RISING_EDGE_EVENT

== stateflow chart Copy_of_minimal_rcu_full/Roboter+controller/controller/Joint Impedance/JOINT_IMPEDANCE_CONTROL/Joint Compliance Control/NAN_checks/hold_zero_if_nan_or_inf8/Hold1 ==
  settings: executeAtInitialization=1
  state OK
    en:error=0;
  state FAIL
    en:error=1;
  (default) -> OK
  OK -> FAIL : isnan
  FAIL -> OK : reset
  data: error output double
  events: isnan input RISING_EDGE_EVENT; reset input RISING_EDGE_EVENT

== matlab function Copy_of_minimal_rcu_full/Roboter+controller/controller/gains_selector/Embedded MATLAB Function ==
  data: BJoint parameter; KT input; B_theta_out output
function B_theta_out  = fcn(BJoint,KT)
% This block supports the Embedded MATLAB subset.
% See the help menu for details. 

B_theta_out= diag(BJoint./(1+KT));
